simulink model "liniarisiert"  (R2015a)
settings: Solver=ode45  StartTime=0.0  StopTime=50  RelTol=1e-3
settings Model: Creator=lustoppe  LastModifiedBy=lustoppe

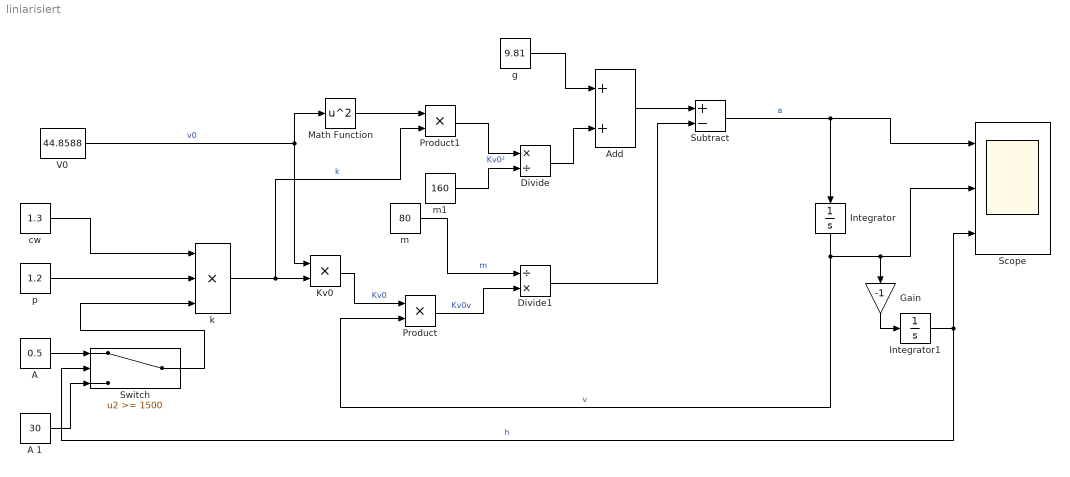
== system liniarisiert ==
  "A " : Constant  Value=0.5
  A 1 : Constant  Value=30
  Add : Sum
  Divide : Product  Inputs=*/
  Divide1 : Product  Inputs=/*
  Gain : Gain  Gain=-1
  Integrator : Integrator
  Integrator1 : Integrator  InitialCondition=3000
  Kv0 : Product
  Math Function : Math  Operator=square  SaturateOnIntegerOverflow=on
  Product : Product
  Product1 : Product
  Scope : Scope  NumInputPorts=3
      settings: YMin=-5~-5~-5  YMax=5~5~5
  Subtract : Sum  Inputs=+-
  Switch : Switch  Threshold=1500
  "V0 " : Constant  Value=44.8588
  "cw " : Constant  Value=1.3
  g : Constant  Value=9.81
  k : Product  Inputs=3
  m : Constant  Value=80
  m1 : Constant  Value=160
  "p " : Constant  Value=1.2
  wires:
  g/1 -> Add/1
  "p "/1 -> k/2
  "cw "/1 -> k/1
  Integrator/1 -> Gain/1, Scope/2, Product/2  "v"
  k/1 -> Product1/2, Kv0/2  "k"
  Kv0/1 -> Product/1  "Kv0"
  Divide/1 -> Add/2
  m/1 -> Divide1/1  "m"
  Product/1 -> Divide1/2  "Kv0v"
  Integrator1/1 -> Scope/3, Switch/2  "h"
  Add/1 -> Subtract/1
  Divide1/1 -> Subtract/2
  "V0 "/1 -> Kv0/1, Math Function/1  "v0"
  Math Function/1 -> Product1/1
  Product1/1 -> Divide/1  "Kv0²"
  m1/1 -> Divide/2
  "A "/1 -> Switch/1
  Switch/1 -> k/3
  A 1/1 -> Switch/3
  Subtract/1 -> Integrator/1, Scope/1  "a"
  Gain/1 -> Integrator1/1
